simulink model "TemplateMatchingCentered"  (R2020a)
settings: Solver=VariableStepAuto  StartTime=0.0  StopTime=10  RelTol=1e-3
undefined symbols (not defined in the file): fs, refractory, th
libraries: simulink x3, dspswit3 x1, dspfdesign x1, hdlsllib x1
settings Model: Creator=sbuccelli  LastModifiedBy=diflo

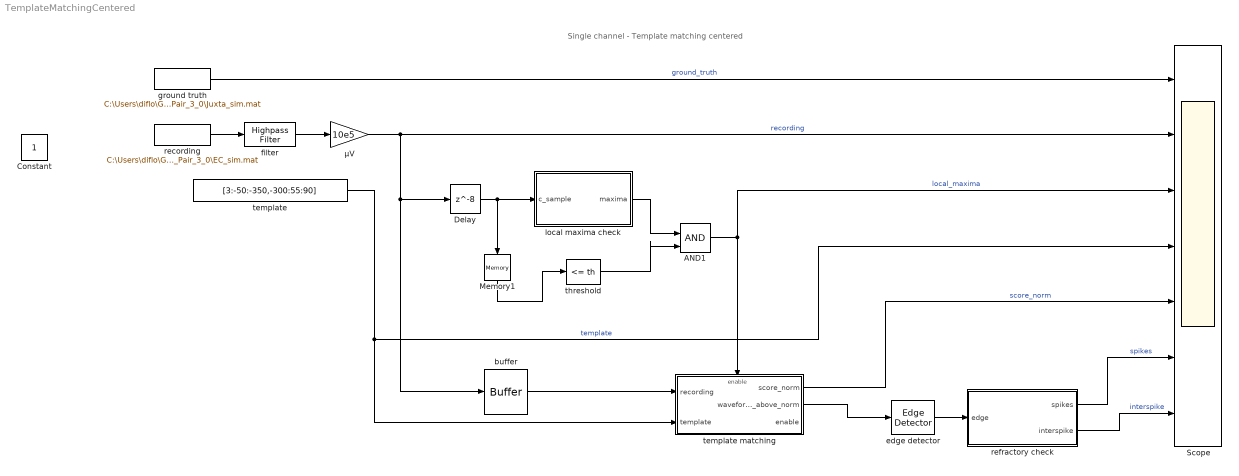
== system TemplateMatchingCentered ==
  note: Single channel - Template matching centered
  AND1 : Logic  IconShape=distinctive  AllPortsSameDT=off
  Delay : Delay  DelayLength=8  InitialCondition=0
  Memory1 : Memory  InheritSampleTime=on
  Scope : Scope  NumInputPorts=7
  buffer : Buffer  N=16  V=15  OutputFrames=off
  edge detector : dspswit3/Edge Detector  InputProcessing=Columns as channels (frame based)
      settings: SourceProductBaseCode=DS
  filter : dspfdesign/Highpass Filter  FilterType=IIR  DesignForMinimumOrder=off  FilterOrder=3  StopbandFrequency=1  PassbandFrequency=300  StopbandAttenuation=80  PassbandRipple=0.1  InheritSampleRate=off  SampleRate=30000  SimulateUsing=Interpreted execution  roundingMode=Floor  coeffsDataTypeStr=fixdt(1,16)
  ground truth : FromFile  FileName=C:\Users\diflo\Google Drive\IIT - Neuroengineering\MathWorks Project\Data\KampffLab\2014_11_25_Pair_3_0\Juxta_sim.mat  SampleTime=1/fs
  local maxima check : Subsystem
  recording : FromFile  FileName=C:\Users\diflo\Google Drive\IIT - Neuroengineering\MathWorks Project\Data\KampffLab\2014_11_25_Pair_3_0\EC_sim.mat  SampleTime=1/fs
  refractory check : Subsystem
  template : Constant  Value=[3:-50:-350,-300:55:90]  SampleTime=1/30000
  template matching : Subsystem
  threshold : simulink/Logic and Bit Operations/Compare To Constant  relop=<=  const=th  OutDataTypeStr=boolean
  μV : Gain  Gain=10e5
  Constant : Constant  IOType=siggen
  wires:
  recording/1 -> filter/1
  filter/1 -> μV/1
  μV/1 -> Scope/2, buffer/1, Delay/1  "recording"
  Delay/1 -> Memory1/1, local maxima check/1(c_sample)
  Memory1/1 -> threshold/1
  local maxima check/1(maxima) -> AND1/1
  threshold/1 -> AND1/2
  AND1/1 -> template matching/Enable, Scope/3  "local_maxima"
  edge detector/1 -> refractory check/1("  edge")
  template matching/2(waveform_above_norm) -> edge detector/1
  buffer/1 -> template matching/1(recording)
  template/1 -> Scope/4, template matching/2(template)  "template"
  ground truth/1 -> Scope/1  "ground_truth"
  template matching/1(score_norm) -> Scope/5  "score_norm"
  refractory check/1(" spikes") -> Scope/6  "spikes"
  refractory check/2(interspike) -> Scope/7  "interspike"

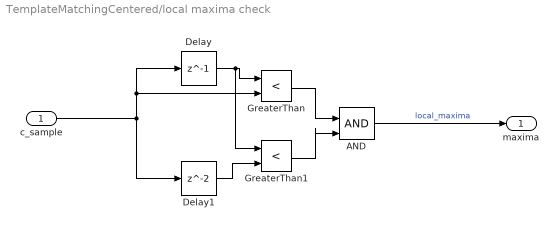
== system TemplateMatchingCentered/local maxima check ==
  c_sample : Inport
  AND : Logic  IconShape=distinctive  AllPortsSameDT=off  OutDataTypeStr=boolean
  Delay : Delay  DelayLength=1  SampleTime=1/30000
  Delay1 : Delay  SampleTime=1/30000
  GreaterThan : RelationalOperator  Operator=<  OutDataTypeStr=boolean  RndMeth=Simplest
  GreaterThan1 : RelationalOperator  Operator=<  OutDataTypeStr=boolean  RndMeth=Simplest
  maxima : Outport
  wires:
  Delay/1 -> GreaterThan1/1, GreaterThan/1
  c_sample/1 -> Delay/1, GreaterThan/2, Delay1/1
  GreaterThan/1 -> AND/1
  GreaterThan1/1 -> AND/2
  AND/1 -> maxima/1  "local_maxima"
  Delay1/1 -> GreaterThan1/2

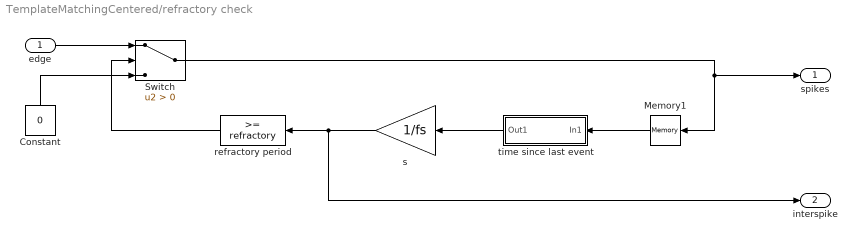
== system TemplateMatchingCentered/refractory check ==
  "  edge" : Inport
  Constant : Constant  Value=0
  Memory1 : Memory  InheritSampleTime=on
  Switch : Switch  Criteria=u2 > Threshold
  refractory period : simulink/Logic and Bit Operations/Compare To Constant  relop=>=  const=refractory  OutDataTypeStr=boolean
  s : Gain  Gain=1/fs  ParamDataTypeStr=double
  time since last event : Subsystem
  " spikes" : Outport
  interspike : Outport  Port=2
  wires:
  "  edge"/1 -> Switch/1
  Memory1/1 -> time since last event/1(In1)
  time since last event/1(Out1) -> s/1
  Constant/1 -> Switch/3
  s/1 -> refractory period/1, interspike/1
  Switch/1 -> " spikes"/1, Memory1/1
  refractory period/1 -> Switch/2

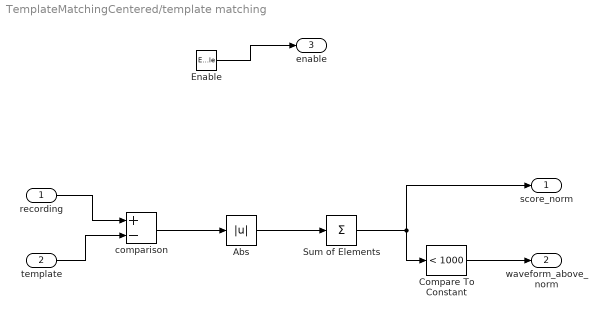
== system TemplateMatchingCentered/template matching ==
  recording : Inport
  template : Inport  Port=2
  Enable : EnablePort  ShowOutputPort=on
  Abs : Abs
  Compare To Constant : simulink/Logic and Bit Operations/Compare To Constant  relop=<  const=1000  OutDataTypeStr=boolean
  Sum of Elements : Sum  Inputs=+
  comparison : Sum  Inputs=+-
  score_norm : Outport
  waveform_above_norm : Outport  Port=2
  enable : Outport  Port=3
  wires:
  Abs/1 -> Sum of Elements/1
  comparison/1 -> Abs/1
  Sum of Elements/1 -> Compare To Constant/1, score_norm/1
  Compare To Constant/1 -> waveform_above_norm/1
  recording/1 -> comparison/1
  template/1 -> comparison/2
  Enable/1 -> enable/1

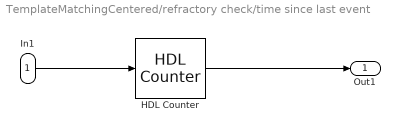
== system TemplateMatchingCentered/refractory check/time since last event ==
  In1 : Inport
  HDL Counter : hdlsllib/Sources/HDL Counter  CountType=Free running  CountInit=1  CountStep=1  CountMax=25  CountFromType=Initial value  CountFrom=1  CountResetPort=on  CountLoadPort=off  CountEnbPort=off  CountDirPort=off  CountDataType=Unsigned  CountWordLen=32  CountFracLen=0  CountSampTime=1
  Out1 : Outport
  wires:
  In1/1 -> HDL Counter/1
  HDL Counter/1 -> Out1/1
